simulink model "sistema_con_reazione_stato"  (R2025b)
settings: Solver=VariableStepAuto  StartTime=0.0  StopTime=20  RelTol=1e-3
undefined symbols (not defined in the file): k1, k2, k3, k4, limite_inf_att, limite_sup_att, ritardo_misura, tau_derivatore, teta_zero, Ts_sens_teta, Ts_sens_x
libraries: cstblocks x4, simulink x2
settings Model: Creator=USER  LastModifiedBy=francesco
settings SolverCC: AlgebraicLoopSolver=TrustRegion
settings DebuggingCC: AlgebraicLoopMsg=none  UnconnectedInputMsg=warning  UnconnectedLineMsg=warning
settings ModelReferenceCC: EnableRefExpFcnMdlSchedulingChecks=on
settings RTWCC: GPUComputeCapability=3.5  DLArmComputeVersion=19.05

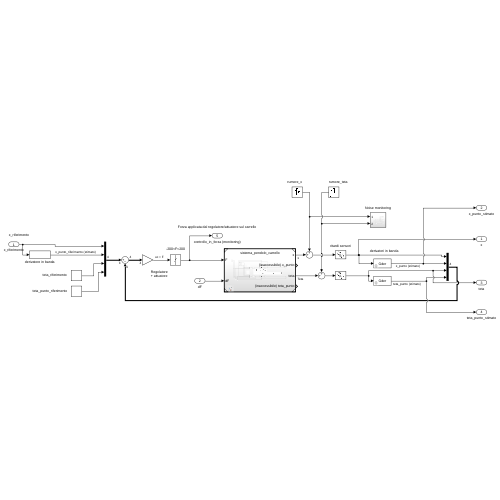
[thumbnail: Simulink's stored preview of the top-level diagram]
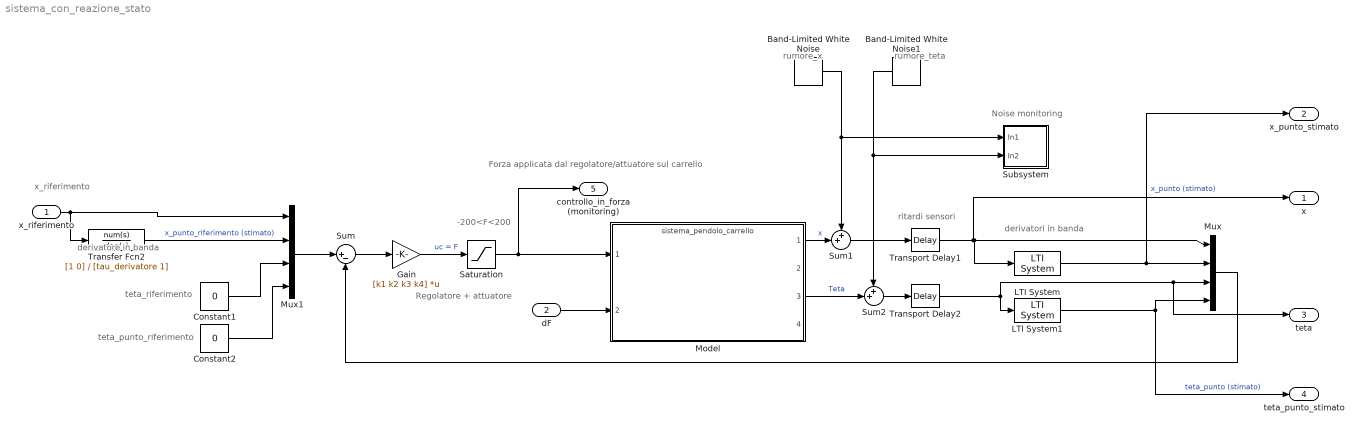
== system sistema_con_reazione_stato ==
  note: Noise monitoring
  note: rumore_teta
  note: rumore_x
  note: derivatore in banda
  note: ritardi sensori
  note: teta_punto_riferimento
  note: teta_riferimento
  note: x_riferimento
  note: derivatori in banda
  note: -200<F<200
  note: Regolatore
      | + attuatore
  note: Forza applicata dal regolatore/attuatore sul carrello
  x_riferimento : Inport
  dF : Inport  Port=2
  Band-Limited White Noise : simulink/Sources/Band-Limited White Noise  Cov=x_noise_power  Ts=Ts_sens_x  seed=[23341]
  Band-Limited White Noise1 : simulink/Sources/Band-Limited White Noise  Cov=teta_noise_power  Ts=Ts_sens_teta  seed=[23341]
  Constant1 : Constant  Value=0
  Constant2 : Constant  Value=0
  Gain : Gain  Gain=[k1 k2 k3 k4]  Multiplication=Matrix(K*u)
  LTI System : cstblocks/LTI System  sys=Gder  IC=[]  PadeOrder=0
  LTI System1 : cstblocks/LTI System  sys=Gder  IC=[]  PadeOrder=0
  Model : ModelReference  ModelNameDialog=sistema_pendolo_carrello.slx  SimulationMode=Normal  ModelReferenceVersion=9.30
  Mux : Mux
  Mux1 : Mux
  Saturation : Saturate  UpperLimit=limite_sup_att  LowerLimit=limite_inf_att
  Subsystem : Subsystem
  Sum : Sum  Inputs=|+-
  Sum1 : Sum  Inputs=++|
  Sum2 : Sum  Inputs=++|
  Transfer Fcn2 : TransferFcn  Numerator=[1 0]  Denominator=[tau_derivatore 1]
  Transport Delay1 : TransportDelay  DelayTime=ritardo_misura
  Transport Delay2 : TransportDelay  DelayTime=ritardo_misura  InitialOutput=teta_zero
  x : Outport
  x_punto_stimato : Outport  Port=2
  teta : Outport  Port=3
  teta_punto_stimato : Outport  Port=4
  controllo_in_forza (monitoring) : Outport  Port=5
  wires:
  Gain/1 -> Saturation/1  "uc = F"
  Saturation/1 -> Model/1, controllo_in_forza (monitoring)/1
  LTI System/1 -> x_punto_stimato/1, Mux/2  "x_punto (stimato)"
  LTI System1/1 -> teta_punto_stimato/1, Mux/4  "teta_punto (stimato)"
  Sum/1 -> Gain/1
  x_riferimento/1 -> Transfer Fcn2/1, Mux1/1
  Constant1/1 -> Mux1/3
  Constant2/1 -> Mux1/4
  Mux1/1 -> Sum/1
  Transfer Fcn2/1 -> Mux1/2  "x_punto_riferimento (stimato)"
  dF/1 -> Model/2
  Mux/1 -> Sum/2
  Transport Delay2/1 -> LTI System1/1, Mux/3, teta/1
  Transport Delay1/1 -> x/1, LTI System/1, Mux/1
  Sum1/1 -> Transport Delay1/1
  Model/1 -> Sum1/2  "x"
  Model/3 -> Sum2/2  "Teta"
  Sum2/1 -> Transport Delay2/1
  Band-Limited White Noise/1 -> Subsystem/1(In1), Sum1/1
  Band-Limited White Noise1/1 -> Subsystem/2(In2), Sum2/1

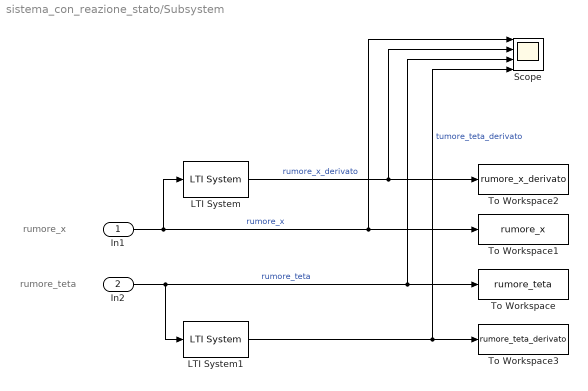
== system sistema_con_reazione_stato/Subsystem ==
  note: rumore_teta
  note: rumore_x
  In1 : Inport
  In2 : Inport  Port=2
  LTI System : cstblocks/LTI System  sys=Gder  IC=[]  PadeOrder=0
  LTI System1 : cstblocks/LTI System  sys=Gder  IC=[]  PadeOrder=0
  Scope : Scope  NumInputPorts=4
      settings: ActiveDisplayString=4  ActiveDisplayYMinimum=-0.020910040248455251  ActiveDisplayYMaximum=0.022610164693865255
  To Workspace : ToWorkspace  VariableName=rumore_teta  SaveFormat=Timeseries  SampleTime=-1
  To Workspace1 : ToWorkspace  VariableName=rumore_x  SaveFormat=Timeseries  SampleTime=-1
  To Workspace2 : ToWorkspace  VariableName=rumore_x_derivato  SaveFormat=Timeseries  SampleTime=-1
  To Workspace3 : ToWorkspace  VariableName=rumore_teta_derivato  SaveFormat=Timeseries  SampleTime=-1
  wires:
  In1/1 -> LTI System/1, To Workspace1/1, Scope/1  "rumore_x"
  LTI System/1 -> To Workspace2/1, Scope/2  "rumore_x_derivato"
  In2/1 -> Scope/3, To Workspace/1, LTI System1/1  "rumore_teta"
  LTI System1/1 -> To Workspace3/1, Scope/4  "tumore_teta_derivato"
